simulink model "main"  (R2015a)
settings: Solver=ode45  StartTime=0.0  StopTime=50  RelTol=1e-3
libraries: simulink x2
settings Model: Creator=jorgeluis  LastModifiedBy=jorgeluis

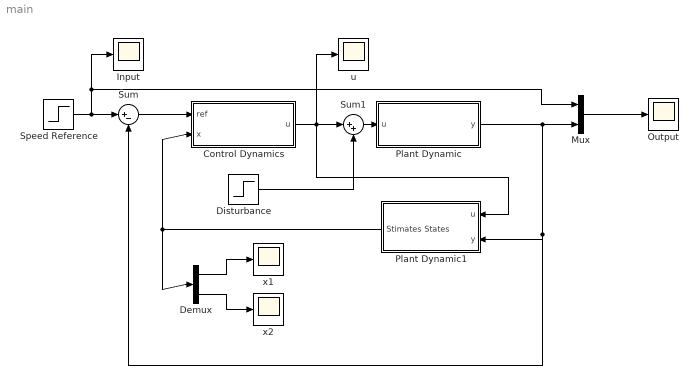
== system main ==
  Control Dynamics : Subsystem
  Demux : Demux  Outputs=2
  Disturbance : Step  Time=200  After=0.1  SampleTime=0
  Input : Scope
      settings: SaveName=ScopeData2
  Mux : Mux  Inputs=2
  Output : Scope
      settings: SaveName=ScopeData3
  Plant Dynamic : Subsystem
  Plant Dynamic1 : Subsystem
  Speed Reference : Step  SampleTime=0
  Sum : Sum  Inputs=|+-
  Sum1 : Sum  Inputs=|++
  u : Scope
      settings: SaveName=ScopeData4
  x1 : Scope
  x2 : Scope
  wires:
  Sum/1 -> Control Dynamics/1(ref)
  Plant Dynamic1/1(Stimates States) -> Control Dynamics/2(x), Demux/1
  Demux/1 -> x1/1
  Demux/2 -> x2/1
  Control Dynamics/1(u) -> u/1, Sum1/1, Plant Dynamic1/1(u)
  Plant Dynamic/1(y) -> Mux/2, Plant Dynamic1/2(y), Sum/2
  Speed Reference/1 -> Mux/1, Input/1, Sum/1
  Mux/1 -> Output/1
  Sum1/1 -> Plant Dynamic/1(u)
  Disturbance/1 -> Sum1/2

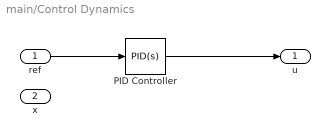
== system main/Control Dynamics ==
  ref : Inport
  x : Inport  Port=2
  PID Controller : simulink/Continuous/PID Controller  Controller=PID  TimeDomain=Continuous-time  SampleTime=-1  IntegratorMethod=Forward Euler  FilterMethod=Forward Euler  Form=Parallel  UseFilter=on  ControllerParametersSource=internal  P=3.09639063366452  I=0.214025276915467  D=1.45626697778434  N=1.4253764986666  InitialConditionSource=internal  InitialConditionForIntegrator=0  InitialConditionForFilter=0  ExternalReset=none  LimitOutput=off  UpperSaturationLimit=inf  LowerSaturationLimit=-inf  LinearizeAsGain=on  AntiWindupMode=none  Kb=1  TrackingMode=off  Kt=1  PParamMin=[]  PParamMax=[]  IParamMin=[]  IParamMax=[]  DParamMin=[]  DParamMax=[]  NParamMin=[]  NParamMax=[]  KbParamMin=[]  KbParamMax=[]  KtParamMin=[]  KtParamMax=[]  POutMin=[]  POutMax=[]  IOutMin=[]  IOutMax=[]  DOutMin=[]  DOutMax=[]  NOutMin=[]  NOutMax=[]  KbOutMin=[]  KbOutMax=[]  KtOutMin=[]  KtOutMax=[]  IntegratorOutMin=[]  IntegratorOutMax=[]  FilterOutMin=[]  FilterOutMax=[]  SumOutMin=[]  SumOutMax=[]  SumI1OutMin=[]  SumI1OutMax=[]  SumI2OutMin=[]  SumI2OutMax=[]  SumI3OutMin=[]  SumI3OutMax=[]  SumDOutMin=[]  SumDOutMax=[]  SaturationOutMin=[]  SaturationOutMax=[]  IntegratorContinuousStateAttributes=''  IntegratorStateMustResolveToSignalObject=off  IntegratorRTWStateStorageClass=Auto  FilterContinuousStateAttributes=''  FilterStateMustResolveToSignalObject=off  FilterRTWStateStorageClass=Auto  DifferentiatorICPrevScaledInput=0  DifferentiatorOutMin=[]  DifferentiatorOutMax=[]
  u : Outport
  wires:
  ref/1 -> PID Controller/1
  PID Controller/1 -> u/1

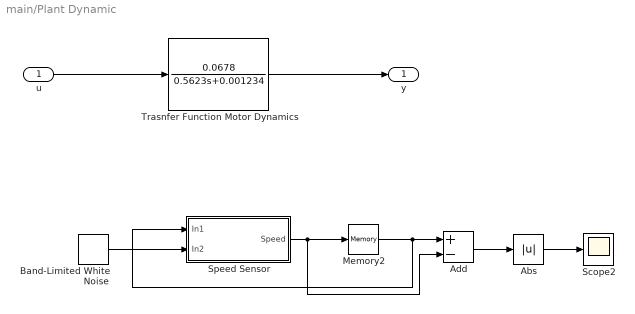
== system main/Plant Dynamic ==
  u : Inport
  Abs : Abs
  Add : Sum  Inputs=+-
  Band-Limited White Noise : simulink/Sources/Band-Limited White Noise  Cov=[0.1]  Ts=0.1  seed=[23341]
  Memory2 : Memory
  Scope2 : Scope
      settings: YMin=0  YMax=275  SaveName=ScopeData5
  Speed Sensor : Subsystem  TreatAsAtomicUnit=on
  Trasnfer Function Motor Dynamics : TransferFcn  Numerator=[0.0678]  Denominator=[0.5623 0.001234]
  y : Outport
  wires:
  u/1 -> Trasnfer Function Motor Dynamics/1
  Trasnfer Function Motor Dynamics/1 -> y/1
  Band-Limited White Noise/1 -> Speed Sensor/2(In2)
  Add/1 -> Abs/1
  Abs/1 -> Scope2/1
  Speed Sensor/1("Speed ") -> Add/2, Memory2/1
  Memory2/1 -> Speed Sensor/1(In1), Add/1

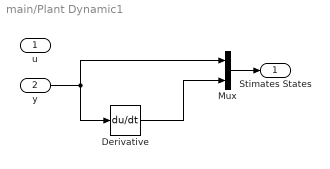
== system main/Plant Dynamic1 ==
  u : Inport
  y : Inport  Port=2
  Derivative : Derivative
  Mux : Mux  Inputs=2
  Stimates States : Outport
  wires:
  Mux/1 -> Stimates States/1
  y/1 -> Derivative/1, Mux/1
  Derivative/1 -> Mux/2

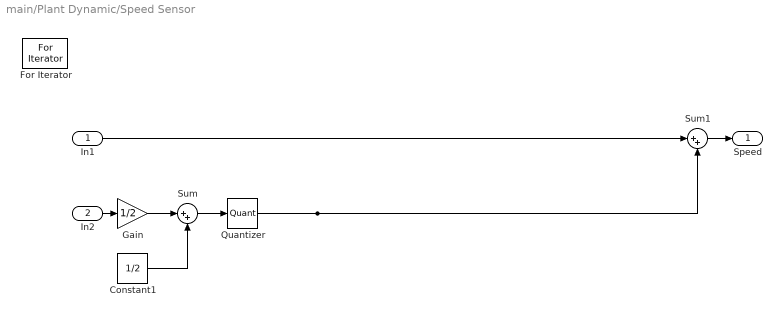
== system main/Plant Dynamic/Speed Sensor ==
  In1 : Inport
  In2 : Inport  Port=2
  Constant1 : Constant  Value=1/2
  For Iterator : ForIterator  IterationLimit=10  IterationVariableDataType=int8
  Gain : Gain  Gain=1/2
  Quantizer : Quantizer  QuantizationInterval=1
  Sum : Sum  Inputs=|++
  Sum1 : Sum  Inputs=|++
  "Speed " : Outport
  wires:
  Constant1/1 -> Sum/2
  In2/1 -> Gain/1
  Gain/1 -> Sum/1
  In1/1 -> Sum1/1
  Sum1/1 -> "Speed "/1
  Sum/1 -> Quantizer/1
  Quantizer/1 -> Sum1/2
